simulink model "TST_CrCtl_Governor"  (R2016b)
settings: Solver=FixedStepDiscrete  StartTime=0.0  StopTime=simTime  FixedStep=sampleTime  RelTol=1e-3
values from neighbouring files (symbols this model uses):
  testCase = 1    [initTST_CrCtl_Governor_001.m]    (also in initTST_CrCtl_Governor_002.m = 2; initTST_CrCtl_Governor_003.m = 3; initTST_CrCtl_Governor_004.m = 4; initTST_CrCtl_Governor_005.m = 5)
libraries: simulink x144, UnitTest_Lib x110
(part 5 of 7)

== system TST_CrCtl_Governor/simulationInput/testSignals_R004 ==
  BC : BusCreator  Inputs=54
  spec_APP_r : FromWorkspace  VariableName=testSig_APP_r  Interpolate=off  OutputAfterFinalValue=Holding final value
  spec_AccPed_trqDes : FromWorkspace  VariableName=testSig_AccPed_trqDes  Interpolate=off  OutputAfterFinalValue=Holding final value
  spec_CoETS_trqNTCActvOff : FromWorkspace  VariableName=testSig_CoETS_trqNTCActvOff  Interpolate=off  OutputAfterFinalValue=Holding final value
  spec_CoETS_trqNTCActvOn : FromWorkspace  VariableName=testSig_CoETS_trqNTCActvOn  Interpolate=off  OutputAfterFinalValue=Holding final value
  spec_CoETS_trqUnFltLtd : FromWorkspace  VariableName=testSig_CoETS_trqUnFltLtd  Interpolate=off  OutputAfterFinalValue=Holding final value
  spec_CoVMD_trqLLim : FromWorkspace  VariableName=testSig_CoVMD_trqLLim  Interpolate=off  OutputAfterFinalValue=Holding final value
  spec_CoVeh_trqAcs : FromWorkspace  VariableName=testSig_CoVeh_trqAcs  Interpolate=off  OutputAfterFinalValue=Holding final value
  spec_CoVeh_trqPrpLimErr : FromWorkspace  VariableName=testSig_CoVeh_trqPrpLimErr  Interpolate=off  OutputAfterFinalValue=Holding final value
  spec_CrCtl_aAccThres : FromWorkspace  VariableName=testSig_CrCtl_aAccThres  Interpolate=off  OutputAfterFinalValue=Holding final value
  spec_CrCtl_aDeclThres : FromWorkspace  VariableName=testSig_CrCtl_aDeclThres  Interpolate=off  OutputAfterFinalValue=Holding final value
  spec_CrCtl_rTraV2NBeg : FromWorkspace  VariableName=testSig_CrCtl_rTraV2NBeg  Interpolate=off  OutputAfterFinalValue=Holding final value
  spec_CrCtl_st : FromWorkspace  VariableName=testSig_CrCtl_st  Interpolate=off  OutputAfterFinalValue=Holding final value
  spec_CrCtl_stGvnr : FromWorkspace  VariableName=testSig_CrCtl_stGvnr  Interpolate=off  OutputAfterFinalValue=Holding final value
  spec_CrCtl_stLck : FromWorkspace  VariableName=testSig_CrCtl_stLck  Interpolate=off  OutputAfterFinalValue=Holding final value
  spec_CrCtl_stOpFunc : FromWorkspace  VariableName=testSig_CrCtl_stOpFunc  Interpolate=off  OutputAfterFinalValue=Holding final value
  spec_CrCtl_stPtd : FromWorkspace  VariableName=testSig_CrCtl_stPtd  Interpolate=off  OutputAfterFinalValue=Holding final value
  spec_CrCtl_stReq : FromWorkspace  VariableName=testSig_CrCtl_stReq  Interpolate=off  OutputAfterFinalValue=Holding final value
  spec_CrCtl_stShOff : FromWorkspace  VariableName=testSig_CrCtl_stShOff  Interpolate=off  OutputAfterFinalValue=Holding final value
  spec_CrCtl_stSub : FromWorkspace  VariableName=testSig_CrCtl_stSub  Interpolate=off  OutputAfterFinalValue=Holding final value
  spec_CrCtl_stSubGvnr : FromWorkspace  VariableName=testSig_CrCtl_stSubGvnr  Interpolate=off  OutputAfterFinalValue=Holding final value
  spec_CrCtl_stSuspAct : FromWorkspace  VariableName=testSig_CrCtl_stSuspAct  Interpolate=off  OutputAfterFinalValue=Holding final value
  spec_CrCtl_stSuspRamp : FromWorkspace  VariableName=testSig_CrCtl_stSuspRamp  Interpolate=off  OutputAfterFinalValue=Holding final value
  spec_CrCtl_stVDirChng : FromWorkspace  VariableName=testSig_CrCtl_stVDirChng  Interpolate=off  OutputAfterFinalValue=Holding final value
  spec_CrCtl_stvHysEngBrkReq : FromWorkspace  VariableName=testSig_CrCtl_stvHysEngBrkReq  Interpolate=off  OutputAfterFinalValue=Holding final value
  spec_CrCtl_trqLead : FromWorkspace  VariableName=testSig_CrCtl_trqLead  Interpolate=off  OutputAfterFinalValue=Holding final value
  spec_CrCtl_trqLimAct : FromWorkspace  VariableName=testSig_CrCtl_trqLimAct  Interpolate=off  OutputAfterFinalValue=Holding final value
  spec_CrCtl_trqMin : FromWorkspace  VariableName=testSig_CrCtl_trqMin  Interpolate=off  OutputAfterFinalValue=Holding final value
  spec_CrCtl_trqReq : FromWorkspace  VariableName=testSig_CrCtl_trqReq  Interpolate=off  OutputAfterFinalValue=Holding final value
  spec_CrCtl_trqReqOld : FromWorkspace  VariableName=testSig_CrCtl_trqReqOld  Interpolate=off  OutputAfterFinalValue=Holding final value
  spec_CrCtl_vDes : FromWorkspace  VariableName=testSig_CrCtl_vDes  Interpolate=off  OutputAfterFinalValue=Holding final value
  spec_CrCtl_vDesAct : FromWorkspace  VariableName=testSig_CrCtl_vDesAct  Interpolate=off  OutputAfterFinalValue=Holding final value
  spec_CrCtl_vDesActOld : FromWorkspace  VariableName=testSig_CrCtl_vDesActOld  Interpolate=off  OutputAfterFinalValue=Holding final value
  spec_CrCtl_vMax : FromWorkspace  VariableName=testSig_CrCtl_vMax  Interpolate=off  OutputAfterFinalValue=Holding final value
  spec_CrCtl_vMaxDvtAcc : FromWorkspace  VariableName=testSig_CrCtl_vMaxDvtAcc  Interpolate=off  OutputAfterFinalValue=Holding final value
  spec_CrCtl_vMaxDvtDecl : FromWorkspace  VariableName=testSig_CrCtl_vMaxDvtDecl  Interpolate=off  OutputAfterFinalValue=Holding final value
  spec_CrCtl_vMin : FromWorkspace  VariableName=testSig_CrCtl_vMin  Interpolate=off  OutputAfterFinalValue=Holding final value
  spec_EBrk_stPreSelMode : FromWorkspace  VariableName=testSig_EBrk_stPreSelMode  Interpolate=off  OutputAfterFinalValue=Holding final value
  spec_EngDem_trqInrLim : FromWorkspace  VariableName=testSig_EngDem_trqInrLim  Interpolate=off  OutputAfterFinalValue=Holding final value
  spec_GlbDa_aXFlt : FromWorkspace  VariableName=testSig_GlbDa_aXFlt  Interpolate=off  OutputAfterFinalValue=Holding final value
  spec_GlbDa_vXFlt : FromWorkspace  VariableName=testSig_GlbDa_vXFlt  Interpolate=off  OutputAfterFinalValue=Holding final value
  spec_InjSys_trqLim : FromWorkspace  VariableName=testSig_InjSys_trqLim  Interpolate=off  OutputAfterFinalValue=Holding final value
  spec_PT_rTraV2N : FromWorkspace  VariableName=testSig_PT_rTraV2N  Interpolate=off  OutputAfterFinalValue=Holding final value
  spec_PT_rTrq : FromWorkspace  VariableName=testSig_PT_rTrq  Interpolate=off  OutputAfterFinalValue=Holding final value
  spec_PT_trqLos : FromWorkspace  VariableName=testSig_PT_trqLos  Interpolate=off  OutputAfterFinalValue=Holding final value
  spec_PT_trqWhl : FromWorkspace  VariableName=testSig_PT_trqWhl  Interpolate=off  OutputAfterFinalValue=Holding final value
  spec_PT_trqWhlMinEng : FromWorkspace  VariableName=testSig_PT_trqWhlMinEng  Interpolate=off  OutputAfterFinalValue=Holding final value
  spec_PT_trqWhlMinEngBrk : FromWorkspace  VariableName=testSig_PT_trqWhlMinEngBrk  Interpolate=off  OutputAfterFinalValue=Holding final value
  spec_RngMod_trqMin : FromWorkspace  VariableName=testSig_RngMod_trqMin  Interpolate=off  OutputAfterFinalValue=Holding final value
  spec_Tra_numGear : FromWorkspace  VariableName=testSig_Tra_numGear  Interpolate=off  OutputAfterFinalValue=Holding final value
  spec_VMD_trqDes : FromWorkspace  VariableName=testSig_VMD_trqDes  Interpolate=off  OutputAfterFinalValue=Holding final value
  spec_VMSAdjBtn_st : FromWorkspace  VariableName=testSig_VMSAdjBtn_st  Interpolate=off  OutputAfterFinalValue=Holding final value
  spec_VMSLmtSwt_st : FromWorkspace  VariableName=testSig_VMSLmtSwt_st  Interpolate=off  OutputAfterFinalValue=Holding final value
  spec_VehMot_rTrqDfftl : FromWorkspace  VariableName=testSig_VehMot_rTrqDfftl  Interpolate=off  OutputAfterFinalValue=Holding final value
  spec_WESDem_stCurr : FromWorkspace  VariableName=testSig_WESDem_stCurr  Interpolate=off  OutputAfterFinalValue=Holding final value
  testSignals : Outport
  wires:
  BC/1 -> testSignals/1
  spec_AccPed_trqDes/1 -> BC/1  "testSig_AccPed_trqDes"
  spec_APP_r/1 -> BC/2  "testSig_APP_r"
  spec_CoETS_trqNTCActvOff/1 -> BC/3  "testSig_CoETS_trqNTCActvOff"
  spec_CoETS_trqNTCActvOn/1 -> BC/4  "testSig_CoETS_trqNTCActvOn"
  spec_CoETS_trqUnFltLtd/1 -> BC/5  "testSig_CoETS_trqUnFltLtd"
  spec_CoVeh_trqAcs/1 -> BC/6  "testSig_CoVeh_trqAcs"
  spec_CoVeh_trqPrpLimErr/1 -> BC/7  "testSig_CoVeh_trqPrpLimErr"
  spec_CoVMD_trqLLim/1 -> BC/8  "testSig_CoVMD_trqLLim"
  spec_CrCtl_aAccThres/1 -> BC/9  "testSig_CrCtl_aAccThres"
  spec_CrCtl_aDeclThres/1 -> BC/10  "testSig_CrCtl_aDeclThres"
  spec_CrCtl_st/1 -> BC/11  "testSig_CrCtl_st"
  spec_CrCtl_stGvnr/1 -> BC/12  "testSig_CrCtl_stGvnr"
  spec_CrCtl_stLck/1 -> BC/13  "testSig_CrCtl_stLck"
  spec_CrCtl_stShOff/1 -> BC/14  "testSig_CrCtl_stShOff"
  spec_CrCtl_stSub/1 -> BC/15  "testSig_CrCtl_stSub"
  spec_CrCtl_stSubGvnr/1 -> BC/16  "testSig_CrCtl_stSubGvnr"
  spec_CrCtl_stSuspAct/1 -> BC/17  "testSig_CrCtl_stSuspAct"
  spec_CrCtl_stVDirChng/1 -> BC/18  "testSig_CrCtl_stVDirChng"
  spec_CrCtl_vDes/1 -> BC/19  "testSig_CrCtl_vDes"
  spec_CrCtl_vDesAct/1 -> BC/20  "testSig_CrCtl_vDesAct"
  spec_CrCtl_vDesActOld/1 -> BC/21  "testSig_CrCtl_vDesActOld"
  spec_CrCtl_vMaxDvtAcc/1 -> BC/22  "testSig_CrCtl_vMaxDvtAcc"
  spec_CrCtl_vMaxDvtDecl/1 -> BC/23  "testSig_CrCtl_vMaxDvtDecl"
  spec_CrCtl_vMin/1 -> BC/24  "testSig_CrCtl_vMin"
  spec_EBrk_stPreSelMode/1 -> BC/25  "testSig_EBrk_stPreSelMode"
  spec_EngDem_trqInrLim/1 -> BC/26  "testSig_EngDem_trqInrLim"
  spec_GlbDa_aXFlt/1 -> BC/27  "testSig_GlbDa_aXFlt"
  spec_GlbDa_vXFlt/1 -> BC/28  "testSig_GlbDa_vXFlt"
  spec_InjSys_trqLim/1 -> BC/29  "testSig_InjSys_trqLim"
  spec_PT_rTraV2N/1 -> BC/30  "testSig_PT_rTraV2N"
  spec_PT_rTrq/1 -> BC/31  "testSig_PT_rTrq"
  spec_PT_trqLos/1 -> BC/32  "testSig_PT_trqLos"
  spec_PT_trqWhl/1 -> BC/33  "testSig_PT_trqWhl"
  spec_PT_trqWhlMinEng/1 -> BC/34  "testSig_PT_trqWhlMinEng"
  spec_PT_trqWhlMinEngBrk/1 -> BC/35  "testSig_PT_trqWhlMinEngBrk"
  spec_RngMod_trqMin/1 -> BC/36  "testSig_RngMod_trqMin"
  spec_Tra_numGear/1 -> BC/37  "testSig_Tra_numGear"
  spec_VehMot_rTrqDfftl/1 -> BC/38  "testSig_VehMot_rTrqDfftl"
  spec_VMD_trqDes/1 -> BC/39  "testSig_VMD_trqDes"
  spec_VMSAdjBtn_st/1 -> BC/40  "testSig_VMSAdjBtn_st"
  spec_VMSLmtSwt_st/1 -> BC/41  "testSig_VMSLmtSwt_st"
  spec_WESDem_stCurr/1 -> BC/42  "testSig_WESDem_stCurr"
  spec_CrCtl_rTraV2NBeg/1 -> BC/43  "testSig_CrCtl_rTraV2NBeg"
  spec_CrCtl_stOpFunc/1 -> BC/44  "testSig_CrCtl_stOpFunc"
  spec_CrCtl_stPtd/1 -> BC/45  "testSig_CrCtl_stPtd"
  spec_CrCtl_stReq/1 -> BC/46  "testSig_CrCtl_stReq"
  spec_CrCtl_stSuspRamp/1 -> BC/47  "testSig_CrCtl_stSuspRamp"
  spec_CrCtl_stvHysEngBrkReq/1 -> BC/48  "testSig_CrCtl_stvHysEngBrkReq"
  spec_CrCtl_trqLead/1 -> BC/49  "testSig_CrCtl_trqLead"
  spec_CrCtl_trqLimAct/1 -> BC/50  "testSig_CrCtl_trqLimAct"
  spec_CrCtl_trqMin/1 -> BC/51  "testSig_CrCtl_trqMin"
  spec_CrCtl_trqReq/1 -> BC/52  "testSig_CrCtl_trqReq"
  spec_CrCtl_trqReqOld/1 -> BC/53  "testSig_CrCtl_trqReqOld"
  spec_CrCtl_vMax/1 -> BC/54  "testSig_CrCtl_vMax"

== system TST_CrCtl_Governor/simulationInput/testSignals_R005 ==
  BC : BusCreator  Inputs=54
  spec_APP_r : FromWorkspace  VariableName=testSig_APP_r  Interpolate=off  OutputAfterFinalValue=Holding final value
  spec_AccPed_trqDes : FromWorkspace  VariableName=testSig_AccPed_trqDes  Interpolate=off  OutputAfterFinalValue=Holding final value
  spec_CoETS_trqNTCActvOff : FromWorkspace  VariableName=testSig_CoETS_trqNTCActvOff  Interpolate=off  OutputAfterFinalValue=Holding final value
  spec_CoETS_trqNTCActvOn : FromWorkspace  VariableName=testSig_CoETS_trqNTCActvOn  Interpolate=off  OutputAfterFinalValue=Holding final value
  spec_CoETS_trqUnFltLtd : FromWorkspace  VariableName=testSig_CoETS_trqUnFltLtd  Interpolate=off  OutputAfterFinalValue=Holding final value
  spec_CoVMD_trqLLim : FromWorkspace  VariableName=testSig_CoVMD_trqLLim  Interpolate=off  OutputAfterFinalValue=Holding final value
  spec_CoVeh_trqAcs : FromWorkspace  VariableName=testSig_CoVeh_trqAcs  Interpolate=off  OutputAfterFinalValue=Holding final value
  spec_CoVeh_trqPrpLimErr : FromWorkspace  VariableName=testSig_CoVeh_trqPrpLimErr  Interpolate=off  OutputAfterFinalValue=Holding final value
  spec_CrCtl_aAccThres : FromWorkspace  VariableName=testSig_CrCtl_aAccThres  Interpolate=off  OutputAfterFinalValue=Holding final value
  spec_CrCtl_aDeclThres : FromWorkspace  VariableName=testSig_CrCtl_aDeclThres  Interpolate=off  OutputAfterFinalValue=Holding final value
  spec_CrCtl_rTraV2NBeg : FromWorkspace  VariableName=testSig_CrCtl_rTraV2NBeg  Interpolate=off  OutputAfterFinalValue=Holding final value
  spec_CrCtl_st : FromWorkspace  VariableName=testSig_CrCtl_st  Interpolate=off  OutputAfterFinalValue=Holding final value
  spec_CrCtl_stGvnr : FromWorkspace  VariableName=testSig_CrCtl_stGvnr  Interpolate=off  OutputAfterFinalValue=Holding final value
  spec_CrCtl_stLck : FromWorkspace  VariableName=testSig_CrCtl_stLck  Interpolate=off  OutputAfterFinalValue=Holding final value
  spec_CrCtl_stOpFunc : FromWorkspace  VariableName=testSig_CrCtl_stOpFunc  Interpolate=off  OutputAfterFinalValue=Holding final value
  spec_CrCtl_stPtd : FromWorkspace  VariableName=testSig_CrCtl_stPtd  Interpolate=off  OutputAfterFinalValue=Holding final value
  spec_CrCtl_stReq : FromWorkspace  VariableName=testSig_CrCtl_stReq  Interpolate=off  OutputAfterFinalValue=Holding final value
  spec_CrCtl_stShOff : FromWorkspace  VariableName=testSig_CrCtl_stShOff  Interpolate=off  OutputAfterFinalValue=Holding final value
  spec_CrCtl_stSub : FromWorkspace  VariableName=testSig_CrCtl_stSub  Interpolate=off  OutputAfterFinalValue=Holding final value
  spec_CrCtl_stSubGvnr : FromWorkspace  VariableName=testSig_CrCtl_stSubGvnr  Interpolate=off  OutputAfterFinalValue=Holding final value
  spec_CrCtl_stSuspAct : FromWorkspace  VariableName=testSig_CrCtl_stSuspAct  Interpolate=off  OutputAfterFinalValue=Holding final value
  spec_CrCtl_stSuspRamp : FromWorkspace  VariableName=testSig_CrCtl_stSuspRamp  Interpolate=off  OutputAfterFinalValue=Holding final value
  spec_CrCtl_stVDirChng : FromWorkspace  VariableName=testSig_CrCtl_stVDirChng  Interpolate=off  OutputAfterFinalValue=Holding final value
  spec_CrCtl_stvHysEngBrkReq : FromWorkspace  VariableName=testSig_CrCtl_stvHysEngBrkReq  Interpolate=off  OutputAfterFinalValue=Holding final value
  spec_CrCtl_trqLead : FromWorkspace  VariableName=testSig_CrCtl_trqLead  Interpolate=off  OutputAfterFinalValue=Holding final value
  spec_CrCtl_trqLimAct : FromWorkspace  VariableName=testSig_CrCtl_trqLimAct  Interpolate=off  OutputAfterFinalValue=Holding final value
  spec_CrCtl_trqMin : FromWorkspace  VariableName=testSig_CrCtl_trqMin  Interpolate=off  OutputAfterFinalValue=Holding final value
  spec_CrCtl_trqReq : FromWorkspace  VariableName=testSig_CrCtl_trqReq  Interpolate=off  OutputAfterFinalValue=Holding final value
  spec_CrCtl_trqReqOld : FromWorkspace  VariableName=testSig_CrCtl_trqReqOld  Interpolate=off  OutputAfterFinalValue=Holding final value
  spec_CrCtl_vDes : FromWorkspace  VariableName=testSig_CrCtl_vDes  Interpolate=off  OutputAfterFinalValue=Holding final value
  spec_CrCtl_vDesAct : FromWorkspace  VariableName=testSig_CrCtl_vDesAct  Interpolate=off  OutputAfterFinalValue=Holding final value
  spec_CrCtl_vDesActOld : FromWorkspace  VariableName=testSig_CrCtl_vDesActOld  Interpolate=off  OutputAfterFinalValue=Holding final value
  spec_CrCtl_vMax : FromWorkspace  VariableName=testSig_CrCtl_vMax  Interpolate=off  OutputAfterFinalValue=Holding final value
  spec_CrCtl_vMaxDvtAcc : FromWorkspace  VariableName=testSig_CrCtl_vMaxDvtAcc  Interpolate=off  OutputAfterFinalValue=Holding final value
  spec_CrCtl_vMaxDvtDecl : FromWorkspace  VariableName=testSig_CrCtl_vMaxDvtDecl  Interpolate=off  OutputAfterFinalValue=Holding final value
  spec_CrCtl_vMin : FromWorkspace  VariableName=testSig_CrCtl_vMin  Interpolate=off  OutputAfterFinalValue=Holding final value
  spec_EBrk_stPreSelMode : FromWorkspace  VariableName=testSig_EBrk_stPreSelMode  Interpolate=off  OutputAfterFinalValue=Holding final value
  spec_EngDem_trqInrLim : FromWorkspace  VariableName=testSig_EngDem_trqInrLim  Interpolate=off  OutputAfterFinalValue=Holding final value
  spec_GlbDa_aXFlt : FromWorkspace  VariableName=testSig_GlbDa_aXFlt  Interpolate=off  OutputAfterFinalValue=Holding final value
  spec_GlbDa_vXFlt : FromWorkspace  VariableName=testSig_GlbDa_vXFlt  Interpolate=off  OutputAfterFinalValue=Holding final value
  spec_InjSys_trqLim : FromWorkspace  VariableName=testSig_InjSys_trqLim  Interpolate=off  OutputAfterFinalValue=Holding final value
  spec_PT_rTraV2N : FromWorkspace  VariableName=testSig_PT_rTraV2N  Interpolate=off  OutputAfterFinalValue=Holding final value
  spec_PT_rTrq : FromWorkspace  VariableName=testSig_PT_rTrq  Interpolate=off  OutputAfterFinalValue=Holding final value
  spec_PT_trqLos : FromWorkspace  VariableName=testSig_PT_trqLos  Interpolate=off  OutputAfterFinalValue=Holding final value
  spec_PT_trqWhl : FromWorkspace  VariableName=testSig_PT_trqWhl  Interpolate=off  OutputAfterFinalValue=Holding final value
  spec_PT_trqWhlMinEng : FromWorkspace  VariableName=testSig_PT_trqWhlMinEng  Interpolate=off  OutputAfterFinalValue=Holding final value
  spec_PT_trqWhlMinEngBrk : FromWorkspace  VariableName=testSig_PT_trqWhlMinEngBrk  Interpolate=off  OutputAfterFinalValue=Holding final value
  spec_RngMod_trqMin : FromWorkspace  VariableName=testSig_RngMod_trqMin  Interpolate=off  OutputAfterFinalValue=Holding final value
  spec_Tra_numGear : FromWorkspace  VariableName=testSig_Tra_numGear  Interpolate=off  OutputAfterFinalValue=Holding final value
  spec_VMD_trqDes : FromWorkspace  VariableName=testSig_VMD_trqDes  Interpolate=off  OutputAfterFinalValue=Holding final value
  spec_VMSAdjBtn_st : FromWorkspace  VariableName=testSig_VMSAdjBtn_st  Interpolate=off  OutputAfterFinalValue=Holding final value
  spec_VMSLmtSwt_st : FromWorkspace  VariableName=testSig_VMSLmtSwt_st  Interpolate=off  OutputAfterFinalValue=Holding final value
  spec_VehMot_rTrqDfftl : FromWorkspace  VariableName=testSig_VehMot_rTrqDfftl  Interpolate=off  OutputAfterFinalValue=Holding final value
  spec_WESDem_stCurr : FromWorkspace  VariableName=testSig_WESDem_stCurr  Interpolate=off  OutputAfterFinalValue=Holding final value
  testSignals : Outport
  wires:
  BC/1 -> testSignals/1
  spec_AccPed_trqDes/1 -> BC/1  "testSig_AccPed_trqDes"
  spec_APP_r/1 -> BC/2  "testSig_APP_r"
  spec_CoETS_trqNTCActvOff/1 -> BC/3  "testSig_CoETS_trqNTCActvOff"
  spec_CoETS_trqNTCActvOn/1 -> BC/4  "testSig_CoETS_trqNTCActvOn"
  spec_CoETS_trqUnFltLtd/1 -> BC/5  "testSig_CoETS_trqUnFltLtd"
  spec_CoVeh_trqAcs/1 -> BC/6  "testSig_CoVeh_trqAcs"
  spec_CoVeh_trqPrpLimErr/1 -> BC/7  "testSig_CoVeh_trqPrpLimErr"
  spec_CoVMD_trqLLim/1 -> BC/8  "testSig_CoVMD_trqLLim"
  spec_CrCtl_aAccThres/1 -> BC/9  "testSig_CrCtl_aAccThres"
  spec_CrCtl_aDeclThres/1 -> BC/10  "testSig_CrCtl_aDeclThres"
  spec_CrCtl_st/1 -> BC/11  "testSig_CrCtl_st"
  spec_CrCtl_stGvnr/1 -> BC/12  "testSig_CrCtl_stGvnr"
  spec_CrCtl_stLck/1 -> BC/13  "testSig_CrCtl_stLck"
  spec_CrCtl_stShOff/1 -> BC/14  "testSig_CrCtl_stShOff"
  spec_CrCtl_stSub/1 -> BC/15  "testSig_CrCtl_stSub"
  spec_CrCtl_stSubGvnr/1 -> BC/16  "testSig_CrCtl_stSubGvnr"
  spec_CrCtl_stSuspAct/1 -> BC/17  "testSig_CrCtl_stSuspAct"
  spec_CrCtl_stVDirChng/1 -> BC/18  "testSig_CrCtl_stVDirChng"
  spec_CrCtl_vDes/1 -> BC/19  "testSig_CrCtl_vDes"
  spec_CrCtl_vDesAct/1 -> BC/20  "testSig_CrCtl_vDesAct"
  spec_CrCtl_vDesActOld/1 -> BC/21  "testSig_CrCtl_vDesActOld"
  spec_CrCtl_vMaxDvtAcc/1 -> BC/22  "testSig_CrCtl_vMaxDvtAcc"
  spec_CrCtl_vMaxDvtDecl/1 -> BC/23  "testSig_CrCtl_vMaxDvtDecl"
  spec_CrCtl_vMin/1 -> BC/24  "testSig_CrCtl_vMin"
  spec_EBrk_stPreSelMode/1 -> BC/25  "testSig_EBrk_stPreSelMode"
  spec_EngDem_trqInrLim/1 -> BC/26  "testSig_EngDem_trqInrLim"
  spec_GlbDa_aXFlt/1 -> BC/27  "testSig_GlbDa_aXFlt"
  spec_GlbDa_vXFlt/1 -> BC/28  "testSig_GlbDa_vXFlt"
  spec_InjSys_trqLim/1 -> BC/29  "testSig_InjSys_trqLim"
  spec_PT_rTraV2N/1 -> BC/30  "testSig_PT_rTraV2N"
  spec_PT_rTrq/1 -> BC/31  "testSig_PT_rTrq"
  spec_PT_trqLos/1 -> BC/32  "testSig_PT_trqLos"
  spec_PT_trqWhl/1 -> BC/33  "testSig_PT_trqWhl"
  spec_PT_trqWhlMinEng/1 -> BC/34  "testSig_PT_trqWhlMinEng"
  spec_PT_trqWhlMinEngBrk/1 -> BC/35  "testSig_PT_trqWhlMinEngBrk"
  spec_RngMod_trqMin/1 -> BC/36  "testSig_RngMod_trqMin"
  spec_Tra_numGear/1 -> BC/37  "testSig_Tra_numGear"
  spec_VehMot_rTrqDfftl/1 -> BC/38  "testSig_VehMot_rTrqDfftl"
  spec_VMD_trqDes/1 -> BC/39  "testSig_VMD_trqDes"
  spec_VMSAdjBtn_st/1 -> BC/40  "testSig_VMSAdjBtn_st"
  spec_VMSLmtSwt_st/1 -> BC/41  "testSig_VMSLmtSwt_st"
  spec_WESDem_stCurr/1 -> BC/42  "testSig_WESDem_stCurr"
  spec_CrCtl_rTraV2NBeg/1 -> BC/43  "testSig_CrCtl_rTraV2NBeg"
  spec_CrCtl_stOpFunc/1 -> BC/44  "testSig_CrCtl_stOpFunc"
  spec_CrCtl_stPtd/1 -> BC/45  "testSig_CrCtl_stPtd"
  spec_CrCtl_stReq/1 -> BC/46  "testSig_CrCtl_stReq"
  spec_CrCtl_stSuspRamp/1 -> BC/47  "testSig_CrCtl_stSuspRamp"
  spec_CrCtl_stvHysEngBrkReq/1 -> BC/48  "testSig_CrCtl_stvHysEngBrkReq"
  spec_CrCtl_trqLead/1 -> BC/49  "testSig_CrCtl_trqLead"
  spec_CrCtl_trqLimAct/1 -> BC/50  "testSig_CrCtl_trqLimAct"
  spec_CrCtl_trqMin/1 -> BC/51  "testSig_CrCtl_trqMin"
  spec_CrCtl_trqReq/1 -> BC/52  "testSig_CrCtl_trqReq"
  spec_CrCtl_trqReqOld/1 -> BC/53  "testSig_CrCtl_trqReqOld"
  spec_CrCtl_vMax/1 -> BC/54  "testSig_CrCtl_vMax"

== system TST_CrCtl_Governor/simulationInput/testSignals_R006 ==
  BC : BusCreator  Inputs=54
  spec_APP_r : FromWorkspace  VariableName=testSig_APP_r  Interpolate=off  OutputAfterFinalValue=Holding final value
  spec_AccPed_trqDes : FromWorkspace  VariableName=testSig_AccPed_trqDes  Interpolate=off  OutputAfterFinalValue=Holding final value
  spec_CoETS_trqNTCActvOff : FromWorkspace  VariableName=testSig_CoETS_trqNTCActvOff  Interpolate=off  OutputAfterFinalValue=Holding final value
  spec_CoETS_trqNTCActvOn : FromWorkspace  VariableName=testSig_CoETS_trqNTCActvOn  Interpolate=off  OutputAfterFinalValue=Holding final value
  spec_CoETS_trqUnFltLtd : FromWorkspace  VariableName=testSig_CoETS_trqUnFltLtd  Interpolate=off  OutputAfterFinalValue=Holding final value
  spec_CoVMD_trqLLim : FromWorkspace  VariableName=testSig_CoVMD_trqLLim  Interpolate=off  OutputAfterFinalValue=Holding final value
  spec_CoVeh_trqAcs : FromWorkspace  VariableName=testSig_CoVeh_trqAcs  Interpolate=off  OutputAfterFinalValue=Holding final value
  spec_CoVeh_trqPrpLimErr : FromWorkspace  VariableName=testSig_CoVeh_trqPrpLimErr  Interpolate=off  OutputAfterFinalValue=Holding final value
  spec_CrCtl_aAccThres : FromWorkspace  VariableName=testSig_CrCtl_aAccThres  Interpolate=off  OutputAfterFinalValue=Holding final value
  spec_CrCtl_aDeclThres : FromWorkspace  VariableName=testSig_CrCtl_aDeclThres  Interpolate=off  OutputAfterFinalValue=Holding final value
  spec_CrCtl_rTraV2NBeg : FromWorkspace  VariableName=testSig_CrCtl_rTraV2NBeg  Interpolate=off  OutputAfterFinalValue=Holding final value
  spec_CrCtl_st : FromWorkspace  VariableName=testSig_CrCtl_st  Interpolate=off  OutputAfterFinalValue=Holding final value
  spec_CrCtl_stGvnr : FromWorkspace  VariableName=testSig_CrCtl_stGvnr  Interpolate=off  OutputAfterFinalValue=Holding final value
  spec_CrCtl_stLck : FromWorkspace  VariableName=testSig_CrCtl_stLck  Interpolate=off  OutputAfterFinalValue=Holding final value
  spec_CrCtl_stOpFunc : FromWorkspace  VariableName=testSig_CrCtl_stOpFunc  Interpolate=off  OutputAfterFinalValue=Holding final value
  spec_CrCtl_stPtd : FromWorkspace  VariableName=testSig_CrCtl_stPtd  Interpolate=off  OutputAfterFinalValue=Holding final value
  spec_CrCtl_stReq : FromWorkspace  VariableName=testSig_CrCtl_stReq  Interpolate=off  OutputAfterFinalValue=Holding final value
  spec_CrCtl_stShOff : FromWorkspace  VariableName=testSig_CrCtl_stShOff  Interpolate=off  OutputAfterFinalValue=Holding final value
  spec_CrCtl_stSub : FromWorkspace  VariableName=testSig_CrCtl_stSub  Interpolate=off  OutputAfterFinalValue=Holding final value
  spec_CrCtl_stSubGvnr : FromWorkspace  VariableName=testSig_CrCtl_stSubGvnr  Interpolate=off  OutputAfterFinalValue=Holding final value
  spec_CrCtl_stSuspAct : FromWorkspace  VariableName=testSig_CrCtl_stSuspAct  Interpolate=off  OutputAfterFinalValue=Holding final value
  spec_CrCtl_stSuspRamp : FromWorkspace  VariableName=testSig_CrCtl_stSuspRamp  Interpolate=off  OutputAfterFinalValue=Holding final value
  spec_CrCtl_stVDirChng : FromWorkspace  VariableName=testSig_CrCtl_stVDirChng  Interpolate=off  OutputAfterFinalValue=Holding final value
  spec_CrCtl_stvHysEngBrkReq : FromWorkspace  VariableName=testSig_CrCtl_stvHysEngBrkReq  Interpolate=off  OutputAfterFinalValue=Holding final value
  spec_CrCtl_trqLead : FromWorkspace  VariableName=testSig_CrCtl_trqLead  Interpolate=off  OutputAfterFinalValue=Holding final value
  spec_CrCtl_trqLimAct : FromWorkspace  VariableName=testSig_CrCtl_trqLimAct  Interpolate=off  OutputAfterFinalValue=Holding final value
  spec_CrCtl_trqMin : FromWorkspace  VariableName=testSig_CrCtl_trqMin  Interpolate=off  OutputAfterFinalValue=Holding final value
  spec_CrCtl_trqReq : FromWorkspace  VariableName=testSig_CrCtl_trqReq  Interpolate=off  OutputAfterFinalValue=Holding final value
  spec_CrCtl_trqReqOld : FromWorkspace  VariableName=testSig_CrCtl_trqReqOld  Interpolate=off  OutputAfterFinalValue=Holding final value
  spec_CrCtl_vDes : FromWorkspace  VariableName=testSig_CrCtl_vDes  Interpolate=off  OutputAfterFinalValue=Holding final value
  spec_CrCtl_vDesAct : FromWorkspace  VariableName=testSig_CrCtl_vDesAct  Interpolate=off  OutputAfterFinalValue=Holding final value
  spec_CrCtl_vDesActOld : FromWorkspace  VariableName=testSig_CrCtl_vDesActOld  Interpolate=off  OutputAfterFinalValue=Holding final value
  spec_CrCtl_vMax : FromWorkspace  VariableName=testSig_CrCtl_vMax  Interpolate=off  OutputAfterFinalValue=Holding final value
  spec_CrCtl_vMaxDvtAcc : FromWorkspace  VariableName=testSig_CrCtl_vMaxDvtAcc  Interpolate=off  OutputAfterFinalValue=Holding final value
  spec_CrCtl_vMaxDvtDecl : FromWorkspace  VariableName=testSig_CrCtl_vMaxDvtDecl  Interpolate=off  OutputAfterFinalValue=Holding final value
  spec_CrCtl_vMin : FromWorkspace  VariableName=testSig_CrCtl_vMin  Interpolate=off  OutputAfterFinalValue=Holding final value
  spec_EBrk_stPreSelMode : FromWorkspace  VariableName=testSig_EBrk_stPreSelMode  Interpolate=off  OutputAfterFinalValue=Holding final value
  spec_EngDem_trqInrLim : FromWorkspace  VariableName=testSig_EngDem_trqInrLim  Interpolate=off  OutputAfterFinalValue=Holding final value
  spec_GlbDa_aXFlt : FromWorkspace  VariableName=testSig_GlbDa_aXFlt  Interpolate=off  OutputAfterFinalValue=Holding final value
  spec_GlbDa_vXFlt : FromWorkspace  VariableName=testSig_GlbDa_vXFlt  Interpolate=off  OutputAfterFinalValue=Holding final value
  spec_InjSys_trqLim : FromWorkspace  VariableName=testSig_InjSys_trqLim  Interpolate=off  OutputAfterFinalValue=Holding final value
  spec_PT_rTraV2N : FromWorkspace  VariableName=testSig_PT_rTraV2N  Interpolate=off  OutputAfterFinalValue=Holding final value
  spec_PT_rTrq : FromWorkspace  VariableName=testSig_PT_rTrq  Interpolate=off  OutputAfterFinalValue=Holding final value
  spec_PT_trqLos : FromWorkspace  VariableName=testSig_PT_trqLos  Interpolate=off  OutputAfterFinalValue=Holding final value
  spec_PT_trqWhl : FromWorkspace  VariableName=testSig_PT_trqWhl  Interpolate=off  OutputAfterFinalValue=Holding final value
  spec_PT_trqWhlMinEng : FromWorkspace  VariableName=testSig_PT_trqWhlMinEng  Interpolate=off  OutputAfterFinalValue=Holding final value
  spec_PT_trqWhlMinEngBrk : FromWorkspace  VariableName=testSig_PT_trqWhlMinEngBrk  Interpolate=off  OutputAfterFinalValue=Holding final value
  spec_RngMod_trqMin : FromWorkspace  VariableName=testSig_RngMod_trqMin  Interpolate=off  OutputAfterFinalValue=Holding final value
  spec_Tra_numGear : FromWorkspace  VariableName=testSig_Tra_numGear  Interpolate=off  OutputAfterFinalValue=Holding final value
  spec_VMD_trqDes : FromWorkspace  VariableName=testSig_VMD_trqDes  Interpolate=off  OutputAfterFinalValue=Holding final value
  spec_VMSAdjBtn_st : FromWorkspace  VariableName=testSig_VMSAdjBtn_st  Interpolate=off  OutputAfterFinalValue=Holding final value
  spec_VMSLmtSwt_st : FromWorkspace  VariableName=testSig_VMSLmtSwt_st  Interpolate=off  OutputAfterFinalValue=Holding final value
  spec_VehMot_rTrqDfftl : FromWorkspace  VariableName=testSig_VehMot_rTrqDfftl  Interpolate=off  OutputAfterFinalValue=Holding final value
  spec_WESDem_stCurr : FromWorkspace  VariableName=testSig_WESDem_stCurr  Interpolate=off  OutputAfterFinalValue=Holding final value
  testSignals : Outport
  wires:
  BC/1 -> testSignals/1
  spec_AccPed_trqDes/1 -> BC/1  "testSig_AccPed_trqDes"
  spec_APP_r/1 -> BC/2  "testSig_APP_r"
  spec_CoETS_trqNTCActvOff/1 -> BC/3  "testSig_CoETS_trqNTCActvOff"
  spec_CoETS_trqNTCActvOn/1 -> BC/4  "testSig_CoETS_trqNTCActvOn"
  spec_CoETS_trqUnFltLtd/1 -> BC/5  "testSig_CoETS_trqUnFltLtd"
  spec_CoVeh_trqAcs/1 -> BC/6  "testSig_CoVeh_trqAcs"
  spec_CoVeh_trqPrpLimErr/1 -> BC/7  "testSig_CoVeh_trqPrpLimErr"
  spec_CoVMD_trqLLim/1 -> BC/8  "testSig_CoVMD_trqLLim"
  spec_CrCtl_aAccThres/1 -> BC/9  "testSig_CrCtl_aAccThres"
  spec_CrCtl_aDeclThres/1 -> BC/10  "testSig_CrCtl_aDeclThres"
  spec_CrCtl_st/1 -> BC/11  "testSig_CrCtl_st"
  spec_CrCtl_stGvnr/1 -> BC/12  "testSig_CrCtl_stGvnr"
  spec_CrCtl_stLck/1 -> BC/13  "testSig_CrCtl_stLck"
  spec_CrCtl_stShOff/1 -> BC/14  "testSig_CrCtl_stShOff"
  spec_CrCtl_stSub/1 -> BC/15  "testSig_CrCtl_stSub"
  spec_CrCtl_stSubGvnr/1 -> BC/16  "testSig_CrCtl_stSubGvnr"
  spec_CrCtl_stSuspAct/1 -> BC/17  "testSig_CrCtl_stSuspAct"
  spec_CrCtl_stVDirChng/1 -> BC/18  "testSig_CrCtl_stVDirChng"
  spec_CrCtl_vDes/1 -> BC/19  "testSig_CrCtl_vDes"
  spec_CrCtl_vDesAct/1 -> BC/20  "testSig_CrCtl_vDesAct"
  spec_CrCtl_vDesActOld/1 -> BC/21  "testSig_CrCtl_vDesActOld"
  spec_CrCtl_vMaxDvtAcc/1 -> BC/22  "testSig_CrCtl_vMaxDvtAcc"
  spec_CrCtl_vMaxDvtDecl/1 -> BC/23  "testSig_CrCtl_vMaxDvtDecl"
  spec_CrCtl_vMin/1 -> BC/24  "testSig_CrCtl_vMin"
  spec_EBrk_stPreSelMode/1 -> BC/25  "testSig_EBrk_stPreSelMode"
  spec_EngDem_trqInrLim/1 -> BC/26  "testSig_EngDem_trqInrLim"
  spec_GlbDa_aXFlt/1 -> BC/27  "testSig_GlbDa_aXFlt"
  spec_GlbDa_vXFlt/1 -> BC/28  "testSig_GlbDa_vXFlt"
  spec_InjSys_trqLim/1 -> BC/29  "testSig_InjSys_trqLim"
  spec_PT_rTraV2N/1 -> BC/30  "testSig_PT_rTraV2N"
  spec_PT_rTrq/1 -> BC/31  "testSig_PT_rTrq"
  spec_PT_trqLos/1 -> BC/32  "testSig_PT_trqLos"
  spec_PT_trqWhl/1 -> BC/33  "testSig_PT_trqWhl"
  spec_PT_trqWhlMinEng/1 -> BC/34  "testSig_PT_trqWhlMinEng"
  spec_PT_trqWhlMinEngBrk/1 -> BC/35  "testSig_PT_trqWhlMinEngBrk"
  spec_RngMod_trqMin/1 -> BC/36  "testSig_RngMod_trqMin"
  spec_Tra_numGear/1 -> BC/37  "testSig_Tra_numGear"
  spec_VehMot_rTrqDfftl/1 -> BC/38  "testSig_VehMot_rTrqDfftl"
  spec_VMD_trqDes/1 -> BC/39  "testSig_VMD_trqDes"
  spec_VMSAdjBtn_st/1 -> BC/40  "testSig_VMSAdjBtn_st"
  spec_VMSLmtSwt_st/1 -> BC/41  "testSig_VMSLmtSwt_st"
  spec_WESDem_stCurr/1 -> BC/42  "testSig_WESDem_stCurr"
  spec_CrCtl_rTraV2NBeg/1 -> BC/43  "testSig_CrCtl_rTraV2NBeg"
  spec_CrCtl_stOpFunc/1 -> BC/44  "testSig_CrCtl_stOpFunc"
  spec_CrCtl_stPtd/1 -> BC/45  "testSig_CrCtl_stPtd"
  spec_CrCtl_stReq/1 -> BC/46  "testSig_CrCtl_stReq"
  spec_CrCtl_stSuspRamp/1 -> BC/47  "testSig_CrCtl_stSuspRamp"
  spec_CrCtl_stvHysEngBrkReq/1 -> BC/48  "testSig_CrCtl_stvHysEngBrkReq"
  spec_CrCtl_trqLead/1 -> BC/49  "testSig_CrCtl_trqLead"
  spec_CrCtl_trqLimAct/1 -> BC/50  "testSig_CrCtl_trqLimAct"
  spec_CrCtl_trqMin/1 -> BC/51  "testSig_CrCtl_trqMin"
  spec_CrCtl_trqReq/1 -> BC/52  "testSig_CrCtl_trqReq"
  spec_CrCtl_trqReqOld/1 -> BC/53  "testSig_CrCtl_trqReqOld"
  spec_CrCtl_vMax/1 -> BC/54  "testSig_CrCtl_vMax"

== system TST_CrCtl_Governor/simulationInput/testSignals_R007 ==
  BC : BusCreator  Inputs=54
  spec_APP_r : FromWorkspace  VariableName=testSig_APP_r  Interpolate=off  OutputAfterFinalValue=Holding final value
  spec_AccPed_trqDes : FromWorkspace  VariableName=testSig_AccPed_trqDes  Interpolate=off  OutputAfterFinalValue=Holding final value
  spec_CoETS_trqNTCActvOff : FromWorkspace  VariableName=testSig_CoETS_trqNTCActvOff  Interpolate=off  OutputAfterFinalValue=Holding final value
  spec_CoETS_trqNTCActvOn : FromWorkspace  VariableName=testSig_CoETS_trqNTCActvOn  Interpolate=off  OutputAfterFinalValue=Holding final value
  spec_CoETS_trqUnFltLtd : FromWorkspace  VariableName=testSig_CoETS_trqUnFltLtd  Interpolate=off  OutputAfterFinalValue=Holding final value
  spec_CoVMD_trqLLim : FromWorkspace  VariableName=testSig_CoVMD_trqLLim  Interpolate=off  OutputAfterFinalValue=Holding final value
  spec_CoVeh_trqAcs : FromWorkspace  VariableName=testSig_CoVeh_trqAcs  Interpolate=off  OutputAfterFinalValue=Holding final value
  spec_CoVeh_trqPrpLimErr : FromWorkspace  VariableName=testSig_CoVeh_trqPrpLimErr  Interpolate=off  OutputAfterFinalValue=Holding final value
  spec_CrCtl_aAccThres : FromWorkspace  VariableName=testSig_CrCtl_aAccThres  Interpolate=off  OutputAfterFinalValue=Holding final value
  spec_CrCtl_aDeclThres : FromWorkspace  VariableName=testSig_CrCtl_aDeclThres  Interpolate=off  OutputAfterFinalValue=Holding final value
  spec_CrCtl_rTraV2NBeg : FromWorkspace  VariableName=testSig_CrCtl_rTraV2NBeg  Interpolate=off  OutputAfterFinalValue=Holding final value
  spec_CrCtl_st : FromWorkspace  VariableName=testSig_CrCtl_st  Interpolate=off  OutputAfterFinalValue=Holding final value
  spec_CrCtl_stGvnr : FromWorkspace  VariableName=testSig_CrCtl_stGvnr  Interpolate=off  OutputAfterFinalValue=Holding final value
  spec_CrCtl_stLck : FromWorkspace  VariableName=testSig_CrCtl_stLck  Interpolate=off  OutputAfterFinalValue=Holding final value
  spec_CrCtl_stOpFunc : FromWorkspace  VariableName=testSig_CrCtl_stOpFunc  Interpolate=off  OutputAfterFinalValue=Holding final value
  spec_CrCtl_stPtd : FromWorkspace  VariableName=testSig_CrCtl_stPtd  Interpolate=off  OutputAfterFinalValue=Holding final value
  spec_CrCtl_stReq : FromWorkspace  VariableName=testSig_CrCtl_stReq  Interpolate=off  OutputAfterFinalValue=Holding final value
  spec_CrCtl_stShOff : FromWorkspace  VariableName=testSig_CrCtl_stShOff  Interpolate=off  OutputAfterFinalValue=Holding final value
  spec_CrCtl_stSub : FromWorkspace  VariableName=testSig_CrCtl_stSub  Interpolate=off  OutputAfterFinalValue=Holding final value
  spec_CrCtl_stSubGvnr : FromWorkspace  VariableName=testSig_CrCtl_stSubGvnr  Interpolate=off  OutputAfterFinalValue=Holding final value
  spec_CrCtl_stSuspAct : FromWorkspace  VariableName=testSig_CrCtl_stSuspAct  Interpolate=off  OutputAfterFinalValue=Holding final value
  spec_CrCtl_stSuspRamp : FromWorkspace  VariableName=testSig_CrCtl_stSuspRamp  Interpolate=off  OutputAfterFinalValue=Holding final value
  spec_CrCtl_stVDirChng : FromWorkspace  VariableName=testSig_CrCtl_stVDirChng  Interpolate=off  OutputAfterFinalValue=Holding final value
  spec_CrCtl_stvHysEngBrkReq : FromWorkspace  VariableName=testSig_CrCtl_stvHysEngBrkReq  Interpolate=off  OutputAfterFinalValue=Holding final value
  spec_CrCtl_trqLead : FromWorkspace  VariableName=testSig_CrCtl_trqLead  Interpolate=off  OutputAfterFinalValue=Holding final value
  spec_CrCtl_trqLimAct : FromWorkspace  VariableName=testSig_CrCtl_trqLimAct  Interpolate=off  OutputAfterFinalValue=Holding final value
  spec_CrCtl_trqMin : FromWorkspace  VariableName=testSig_CrCtl_trqMin  Interpolate=off  OutputAfterFinalValue=Holding final value
  spec_CrCtl_trqReq : FromWorkspace  VariableName=testSig_CrCtl_trqReq  Interpolate=off  OutputAfterFinalValue=Holding final value
  spec_CrCtl_trqReqOld : FromWorkspace  VariableName=testSig_CrCtl_trqReqOld  Interpolate=off  OutputAfterFinalValue=Holding final value
  spec_CrCtl_vDes : FromWorkspace  VariableName=testSig_CrCtl_vDes  Interpolate=off  OutputAfterFinalValue=Holding final value
  spec_CrCtl_vDesAct : FromWorkspace  VariableName=testSig_CrCtl_vDesAct  Interpolate=off  OutputAfterFinalValue=Holding final value
  spec_CrCtl_vDesActOld : FromWorkspace  VariableName=testSig_CrCtl_vDesActOld  Interpolate=off  OutputAfterFinalValue=Holding final value
  spec_CrCtl_vMax : FromWorkspace  VariableName=testSig_CrCtl_vMax  Interpolate=off  OutputAfterFinalValue=Holding final value
  spec_CrCtl_vMaxDvtAcc : FromWorkspace  VariableName=testSig_CrCtl_vMaxDvtAcc  Interpolate=off  OutputAfterFinalValue=Holding final value
  spec_CrCtl_vMaxDvtDecl : FromWorkspace  VariableName=testSig_CrCtl_vMaxDvtDecl  Interpolate=off  OutputAfterFinalValue=Holding final value
  spec_CrCtl_vMin : FromWorkspace  VariableName=testSig_CrCtl_vMin  Interpolate=off  OutputAfterFinalValue=Holding final value
  spec_EBrk_stPreSelMode : FromWorkspace  VariableName=testSig_EBrk_stPreSelMode  Interpolate=off  OutputAfterFinalValue=Holding final value
  spec_EngDem_trqInrLim : FromWorkspace  VariableName=testSig_EngDem_trqInrLim  Interpolate=off  OutputAfterFinalValue=Holding final value
  spec_GlbDa_aXFlt : FromWorkspace  VariableName=testSig_GlbDa_aXFlt  Interpolate=off  OutputAfterFinalValue=Holding final value
  spec_GlbDa_vXFlt : FromWorkspace  VariableName=testSig_GlbDa_vXFlt  Interpolate=off  OutputAfterFinalValue=Holding final value
  spec_InjSys_trqLim : FromWorkspace  VariableName=testSig_InjSys_trqLim  Interpolate=off  OutputAfterFinalValue=Holding final value
  spec_PT_rTraV2N : FromWorkspace  VariableName=testSig_PT_rTraV2N  Interpolate=off  OutputAfterFinalValue=Holding final value
  spec_PT_rTrq : FromWorkspace  VariableName=testSig_PT_rTrq  Interpolate=off  OutputAfterFinalValue=Holding final value
  spec_PT_trqLos : FromWorkspace  VariableName=testSig_PT_trqLos  Interpolate=off  OutputAfterFinalValue=Holding final value
  spec_PT_trqWhl : FromWorkspace  VariableName=testSig_PT_trqWhl  Interpolate=off  OutputAfterFinalValue=Holding final value
  spec_PT_trqWhlMinEng : FromWorkspace  VariableName=testSig_PT_trqWhlMinEng  Interpolate=off  OutputAfterFinalValue=Holding final value
  spec_PT_trqWhlMinEngBrk : FromWorkspace  VariableName=testSig_PT_trqWhlMinEngBrk  Interpolate=off  OutputAfterFinalValue=Holding final value
  spec_RngMod_trqMin : FromWorkspace  VariableName=testSig_RngMod_trqMin  Interpolate=off  OutputAfterFinalValue=Holding final value
  spec_Tra_numGear : FromWorkspace  VariableName=testSig_Tra_numGear  Interpolate=off  OutputAfterFinalValue=Holding final value
  spec_VMD_trqDes : FromWorkspace  VariableName=testSig_VMD_trqDes  Interpolate=off  OutputAfterFinalValue=Holding final value
  spec_VMSAdjBtn_st : FromWorkspace  VariableName=testSig_VMSAdjBtn_st  Interpolate=off  OutputAfterFinalValue=Holding final value
  spec_VMSLmtSwt_st : FromWorkspace  VariableName=testSig_VMSLmtSwt_st  Interpolate=off  OutputAfterFinalValue=Holding final value
  spec_VehMot_rTrqDfftl : FromWorkspace  VariableName=testSig_VehMot_rTrqDfftl  Interpolate=off  OutputAfterFinalValue=Holding final value
  spec_WESDem_stCurr : FromWorkspace  VariableName=testSig_WESDem_stCurr  Interpolate=off  OutputAfterFinalValue=Holding final value
  testSignals : Outport
  wires:
  BC/1 -> testSignals/1
  spec_AccPed_trqDes/1 -> BC/1  "testSig_AccPed_trqDes"
  spec_APP_r/1 -> BC/2  "testSig_APP_r"
  spec_CoETS_trqNTCActvOff/1 -> BC/3  "testSig_CoETS_trqNTCActvOff"
  spec_CoETS_trqNTCActvOn/1 -> BC/4  "testSig_CoETS_trqNTCActvOn"
  spec_CoETS_trqUnFltLtd/1 -> BC/5  "testSig_CoETS_trqUnFltLtd"
  spec_CoVeh_trqAcs/1 -> BC/6  "testSig_CoVeh_trqAcs"
  spec_CoVeh_trqPrpLimErr/1 -> BC/7  "testSig_CoVeh_trqPrpLimErr"
  spec_CoVMD_trqLLim/1 -> BC/8  "testSig_CoVMD_trqLLim"
  spec_CrCtl_aAccThres/1 -> BC/9  "testSig_CrCtl_aAccThres"
  spec_CrCtl_aDeclThres/1 -> BC/10  "testSig_CrCtl_aDeclThres"
  spec_CrCtl_st/1 -> BC/11  "testSig_CrCtl_st"
  spec_CrCtl_stGvnr/1 -> BC/12  "testSig_CrCtl_stGvnr"
  spec_CrCtl_stLck/1 -> BC/13  "testSig_CrCtl_stLck"
  spec_CrCtl_stShOff/1 -> BC/14  "testSig_CrCtl_stShOff"
  spec_CrCtl_stSub/1 -> BC/15  "testSig_CrCtl_stSub"
  spec_CrCtl_stSubGvnr/1 -> BC/16  "testSig_CrCtl_stSubGvnr"
  spec_CrCtl_stSuspAct/1 -> BC/17  "testSig_CrCtl_stSuspAct"
  spec_CrCtl_stVDirChng/1 -> BC/18  "testSig_CrCtl_stVDirChng"
  spec_CrCtl_vDes/1 -> BC/19  "testSig_CrCtl_vDes"
  spec_CrCtl_vDesAct/1 -> BC/20  "testSig_CrCtl_vDesAct"
  spec_CrCtl_vDesActOld/1 -> BC/21  "testSig_CrCtl_vDesActOld"
  spec_CrCtl_vMaxDvtAcc/1 -> BC/22  "testSig_CrCtl_vMaxDvtAcc"
  spec_CrCtl_vMaxDvtDecl/1 -> BC/23  "testSig_CrCtl_vMaxDvtDecl"
  spec_CrCtl_vMin/1 -> BC/24  "testSig_CrCtl_vMin"
  spec_EBrk_stPreSelMode/1 -> BC/25  "testSig_EBrk_stPreSelMode"
  spec_EngDem_trqInrLim/1 -> BC/26  "testSig_EngDem_trqInrLim"
  spec_GlbDa_aXFlt/1 -> BC/27  "testSig_GlbDa_aXFlt"
  spec_GlbDa_vXFlt/1 -> BC/28  "testSig_GlbDa_vXFlt"
  spec_InjSys_trqLim/1 -> BC/29  "testSig_InjSys_trqLim"
  spec_PT_rTraV2N/1 -> BC/30  "testSig_PT_rTraV2N"
  spec_PT_rTrq/1 -> BC/31  "testSig_PT_rTrq"
  spec_PT_trqLos/1 -> BC/32  "testSig_PT_trqLos"
  spec_PT_trqWhl/1 -> BC/33  "testSig_PT_trqWhl"
  spec_PT_trqWhlMinEng/1 -> BC/34  "testSig_PT_trqWhlMinEng"
  spec_PT_trqWhlMinEngBrk/1 -> BC/35  "testSig_PT_trqWhlMinEngBrk"
  spec_RngMod_trqMin/1 -> BC/36  "testSig_RngMod_trqMin"
  spec_Tra_numGear/1 -> BC/37  "testSig_Tra_numGear"
  spec_VehMot_rTrqDfftl/1 -> BC/38  "testSig_VehMot_rTrqDfftl"
  spec_VMD_trqDes/1 -> BC/39  "testSig_VMD_trqDes"
  spec_VMSAdjBtn_st/1 -> BC/40  "testSig_VMSAdjBtn_st"
  spec_VMSLmtSwt_st/1 -> BC/41  "testSig_VMSLmtSwt_st"
  spec_WESDem_stCurr/1 -> BC/42  "testSig_WESDem_stCurr"
  spec_CrCtl_rTraV2NBeg/1 -> BC/43  "testSig_CrCtl_rTraV2NBeg"
  spec_CrCtl_stOpFunc/1 -> BC/44  "testSig_CrCtl_stOpFunc"
  spec_CrCtl_stPtd/1 -> BC/45  "testSig_CrCtl_stPtd"
  spec_CrCtl_stReq/1 -> BC/46  "testSig_CrCtl_stReq"
  spec_CrCtl_stSuspRamp/1 -> BC/47  "testSig_CrCtl_stSuspRamp"
  spec_CrCtl_stvHysEngBrkReq/1 -> BC/48  "testSig_CrCtl_stvHysEngBrkReq"
  spec_CrCtl_trqLead/1 -> BC/49  "testSig_CrCtl_trqLead"
  spec_CrCtl_trqLimAct/1 -> BC/50  "testSig_CrCtl_trqLimAct"
  spec_CrCtl_trqMin/1 -> BC/51  "testSig_CrCtl_trqMin"
  spec_CrCtl_trqReq/1 -> BC/52  "testSig_CrCtl_trqReq"
  spec_CrCtl_trqReqOld/1 -> BC/53  "testSig_CrCtl_trqReqOld"
  spec_CrCtl_vMax/1 -> BC/54  "testSig_CrCtl_vMax"
